simulink model "Senior_Design_G4"  (R2017b)
settings: Solver=ode3  StartTime=0.0  StopTime=inf  FixedStep=0.001  RelTol=1e-3  EnableMultiTasking=on
libraries: xpcquanserlib x5, slrtlib x2
settings Model: SimulationMode=external  Creator=Ninad  LastModifiedBy=basil
settings DataIOCC: LimitDataPoints=on  SaveFormat=Array
settings OptimizationCC: BlockReduction=off  OptimizeBlockIOStorage=off  BufferReuse=off  GlobalBufferReuse=off  ExpressionFolding=off  ExpressionDepthLimit=2147483647  LocalBlockOutputs=off  LifeSpan=inf
settings DebuggingCC: UnderspecifiedInitializationDetection=Classic  MergeDetectMultiDrivingBlocksExec=none  SolverPrmCheckMsg=warning  FcnCallInpInsideContextMsg=warning  StateNameClashWarn=warning  StrictBusMsg=Warning  SFUnexpectedBacktrackingDiag=warning  SFNoUnconditionalDefaultTransitionDiag=warning  SFExecutionAtInitializationDiag=none
settings HardwareCC: ProdBitPerPointer=32  ProdBitPerSizeT=32  ProdBitPerPtrDiffT=32  ProdLargestAtomicFloat=None  ProdWordSize=32  ProdLongLongMode=on  ProdHWDeviceType=Generic->32-bit x86 compatible
settings ModelReferenceCC: PropagateSignalLabelsOutOfModel=off
settings RTWCC: SystemTargetFile=slrt.tlc  TemplateMakefile=slrt_default_tmf  Description=Simulink Real-Time  CodeExecutionProfiling=on  RTWCompilerOptimization=on
settings CodeAppCC: StateflowObjectComments=on
settings SimulinkRealTimeCC: GeneratePreprocessorConditionals=Disable all
settings ConfigComp: CovMetricSettings=dw  CovHtmlReporting=on  CovSaveCumulativeToWorkspaceVar=on  CovSaveSingleToWorkspaceVar=on  CovExternalEMLEnable=off  CovSFcnEnable=off

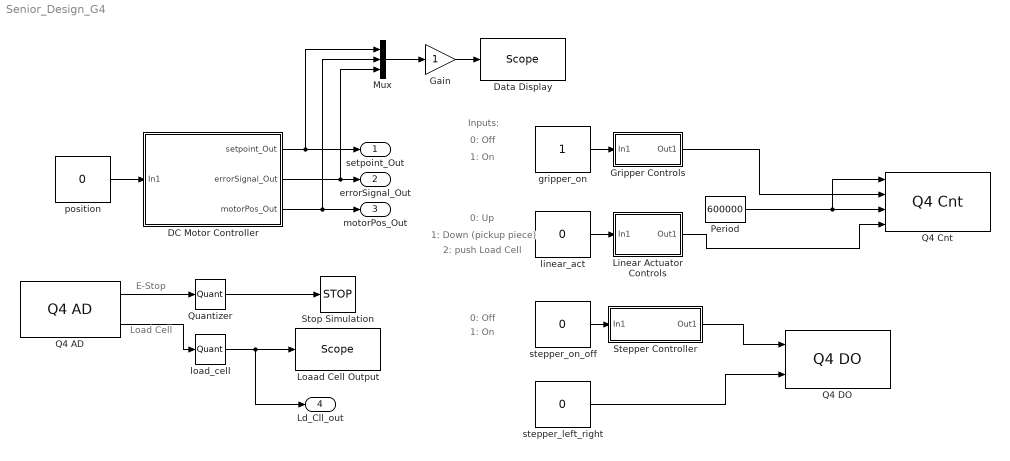
== system Senior_Design_G4 ==
  note: 1: On
  note: 0: Off
  note: 2: push Load Cell
  note: 1: Down (pickup piece)
  note: 0: Up
  note: 1: On
  note: 0: Off
  note: Inputs:
  note: Load Cell
  note: E-Stop
  DC Motor Controller : Subsystem
  Data Display : slrtlib/Displays and Logging/Scope   scopeno=1  scopetype=Target  autostart=on  viewmode=Numerical  formatstr="'Setpoint        %3.2f,Motor Position  %3.2f,Error Signal    %3.2f'"  grid=on  ylimits=[0,170]  nosamples=200  noprepostsamples=0  interleave=10  triggermode=FreeRun  triggersignal=1  trigsignalfromport=off  triggerlevel=0.0  triggerslope=Either  triggerscope=1  triggersample=0  filename=data.dat  mode=Lazy  writesize=512  autorestart=off  dynamicfilemode=off  maxwritefilesize=512*1024^2
  Gain : Gain
  Gripper Controls : Subsystem
  Linear Actuator Controls : Subsystem
  "Loaad Cell Output " : slrtlib/Displays and Logging/Scope   scopeno=4  scopetype=Target  autostart=on  viewmode=Graphical rolling  formatstr='%15.6f'  grid=on  ylimits=[-1,6]  nosamples=500  noprepostsamples=0  interleave=1  triggermode=FreeRun  triggersignal=1  trigsignalfromport=off  triggerlevel=0.0  triggerslope=Either  triggerscope=1  triggersample=0  filename=data.dat  mode=Lazy  writesize=512  autorestart=off  dynamicfilemode=off  maxwritefilesize=512*1024^2
  Mux : Mux  Inputs=3
  Period : Constant  Value=600000
  Q4 AD : xpcquanserlib/A//D/Q4 AD  channel=[1:2]  sampleTime=0.001  slot=-1
      settings: SourceProductName=Simulink Real-Time  SourceProductBaseCode=XP
  "Q4 Cnt " : xpcquanserlib/Counter/Q4 Cnt   channel=[1:2]  mode=[1]  showArm=[0]  reset=[1]  initLoCount=[0]  initHiCount=[0]  sampleTime=.001  slot=-1
      settings: SourceProductName=Simulink Real-Time  SourceProductBaseCode=XP
  "Q4 DO " : xpcquanserlib/Digital Output/Q4 DO   channel=[1:2]  reset=[1]  initValue=[0]  sampleTime=.001  slot=-1
      settings: SourceProductName=Simulink Real-Time  SourceProductBaseCode=XP
  Quantizer : Quantizer  QuantizationInterval=1
  Stepper Controller : Subsystem
  Stop Simulation : Stop
  gripper_on : Constant
  linear_act : Constant  Value=0
  load_cell : Quantizer  QuantizationInterval=5
  position : Constant  Value=0
  stepper_left_right : Constant  Value=0
  stepper_on_off : Constant  Value=0
  setpoint_Out : Outport
  errorSignal_Out : Outport  Port=2
  motorPos_Out : Outport  Port=3
  Ld_Cll_out : Outport  Port=4
  wires:
  Quantizer/1 -> Stop Simulation/1
  Q4 AD/1 -> Quantizer/1
  Q4 AD/2 -> load_cell/1
  load_cell/1 -> Ld_Cll_out/1, "Loaad Cell Output "/1
  Period/1 -> "Q4 Cnt "/1, "Q4 Cnt "/3
  stepper_left_right/1 -> "Q4 DO "/2
  DC Motor Controller/3(motorPos_Out) -> Mux/2, motorPos_Out/1
  position/1 -> DC Motor Controller/1(In1)
  gripper_on/1 -> Gripper Controls/1(In1)
  Gripper Controls/1(Out1) -> "Q4 Cnt "/2
  linear_act/1 -> Linear Actuator Controls/1(In1)
  Linear Actuator Controls/1(Out1) -> "Q4 Cnt "/4
  stepper_on_off/1 -> Stepper Controller/1(In1)
  Stepper Controller/1(Out1) -> "Q4 DO "/1
  Gain/1 -> Data Display/1
  DC Motor Controller/1(setpoint_Out) -> Mux/1, setpoint_Out/1
  DC Motor Controller/2(errorSignal_Out) -> Mux/3, errorSignal_Out/1
  Mux/1 -> Gain/1

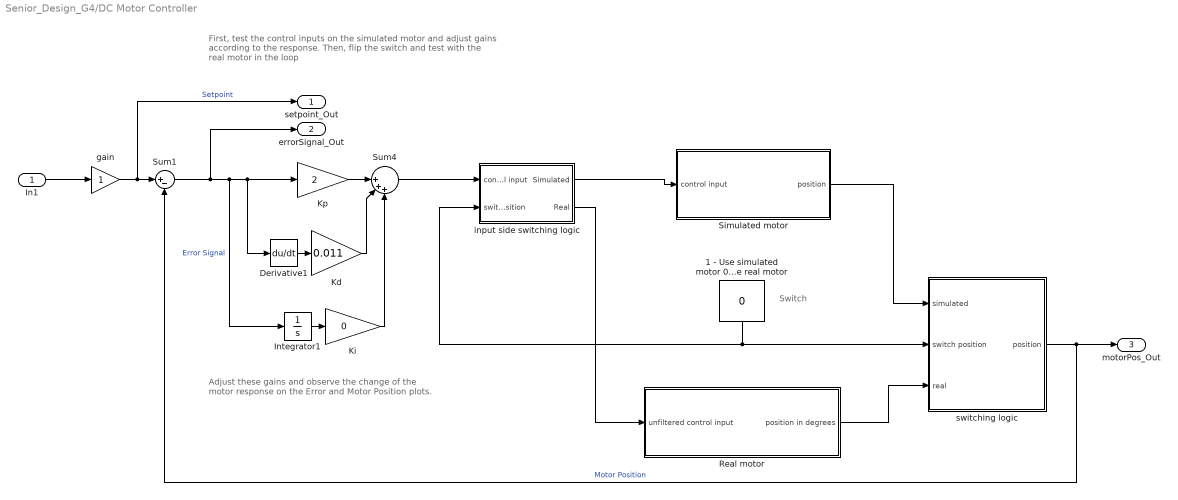
== system Senior_Design_G4/DC Motor Controller ==
  note: Adjust these gains and observe the change of the
      | motor response on the Error and Motor Position
      | plots.
  note: First, test the control inputs on the simulated motor and
      | adjust gains according to the response. Then, flip the switch and
      | test with the real motor in the loop
  note: Switch
  In1 : Inport
  1 - Use simulated motor 0 - Use real motor : Constant  Value=0
  Derivative1 : Derivative
  Integrator1 : Integrator
  Kd : Gain  Gain=0.011
  Ki : Gain  Gain=0
  Kp : Gain  Gain=2
  Real motor : Subsystem
  Simulated motor : Subsystem
  Sum1 : Sum  Inputs=|+-
  Sum4 : Sum  Inputs=||+++
  gain : Gain
  input side switching logic : Subsystem
  switching logic : Subsystem
  setpoint_Out : Outport
  errorSignal_Out : Outport  Port=2
  motorPos_Out : Outport  Port=3
  wires:
  Kp/1 -> Sum4/1
  Kd/1 -> Sum4/2
  Derivative1/1 -> Kd/1
  Ki/1 -> Sum4/3
  Integrator1/1 -> Ki/1
  Sum1/1 -> Kp/1, Derivative1/1, Integrator1/1, errorSignal_Out/1  "Error Signal"
  Simulated motor/1(position) -> switching logic/1(simulated)
  Real motor/1(position in degrees) -> switching logic/3(real)
  switching logic/1(position) -> motorPos_Out/1, Sum1/2  "Motor Position"
  Sum4/1 -> input side switching logic/1(control input)
  input side switching logic/1(Simulated) -> Simulated motor/1(control input)
  input side switching logic/2(Real) -> Real motor/1(unfiltered control input)
  1 - Use simulated motor 0 - Use real motor/1 -> switching logic/2(switch position), input side switching logic/2(switch position)
  In1/1 -> gain/1
  gain/1 -> Sum1/1, setpoint_Out/1  "Setpoint"

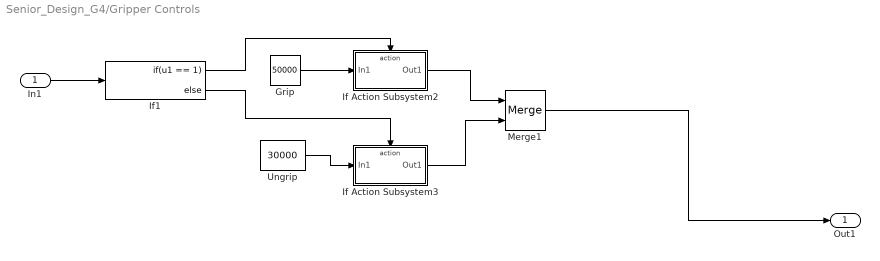
== system Senior_Design_G4/Gripper Controls ==
  In1 : Inport
  Grip : Constant  Value=50000
  If Action Subsystem2 : Subsystem  TreatAsAtomicUnit=on
  If Action Subsystem3 : Subsystem  TreatAsAtomicUnit=on
  If1 : If  IfExpression=u1 == 1
  Merge1 : Merge
  Ungrip : Constant  Value=30000
  Out1 : Outport
  wires:
  If Action Subsystem3/1(Out1) -> Merge1/2
  If Action Subsystem2/1(Out1) -> Merge1/1
  If1/2 -> If Action Subsystem3/Action
  Merge1/1 -> Out1/1
  If1/1 -> If Action Subsystem2/Action
  Grip/1 -> If Action Subsystem2/1(In1)
  In1/1 -> If1/1
  Ungrip/1 -> If Action Subsystem3/1(In1)

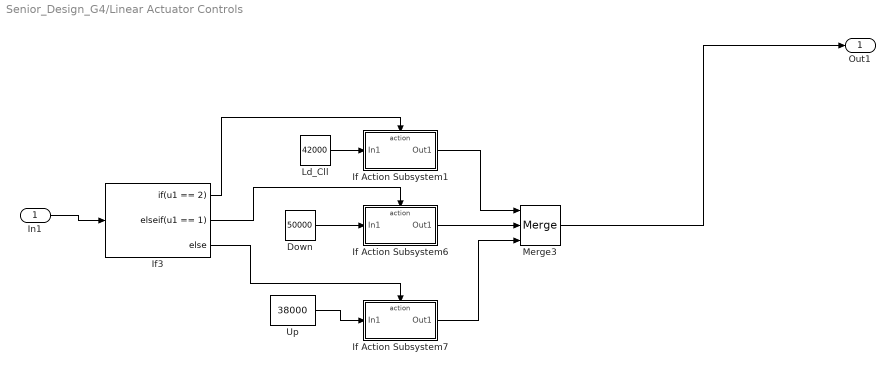
== system Senior_Design_G4/Linear Actuator Controls ==
  In1 : Inport
  Down : Constant  Value=50000
  If Action Subsystem1 : Subsystem  TreatAsAtomicUnit=on
  If Action Subsystem6 : Subsystem  TreatAsAtomicUnit=on
  If Action Subsystem7 : Subsystem  TreatAsAtomicUnit=on
  If3 : If  IfExpression=u1 == 2  ElseIfExpressions=u1 == 1
  Ld_Cll : Constant  Value=42000
  Merge3 : Merge  Inputs=3
  "Up " : Constant  Value=38000
  Out1 : Outport
  wires:
  If Action Subsystem7/1(Out1) -> Merge3/3
  Ld_Cll/1 -> If Action Subsystem1/1(In1)
  "Up "/1 -> If Action Subsystem7/1(In1)
  If3/1 -> If Action Subsystem1/Action
  If3/2 -> If Action Subsystem6/Action
  If3/3 -> If Action Subsystem7/Action
  Down/1 -> If Action Subsystem6/1(In1)
  If Action Subsystem1/1(Out1) -> Merge3/1
  In1/1 -> If3/1
  Merge3/1 -> Out1/1
  If Action Subsystem6/1(Out1) -> Merge3/2

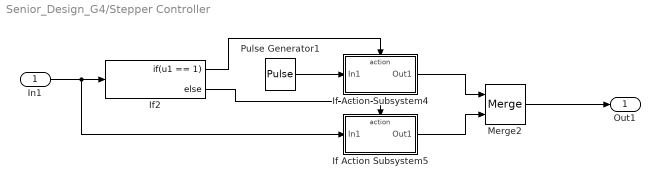
== system Senior_Design_G4/Stepper Controller ==
  In1 : Inport
  If Action Subsystem4 : Subsystem  TreatAsAtomicUnit=on
  If Action Subsystem5 : Subsystem  TreatAsAtomicUnit=on
  If2 : If  IfExpression=u1 == 1
  Merge2 : Merge
  Pulse Generator1 : DiscretePulseGenerator  PulseType=Time based  Amplitude=5  Period=0.01  PulseWidth=50
  Out1 : Outport
  wires:
  In1/1 -> If Action Subsystem5/1(In1), If2/1
  If2/1 -> If Action Subsystem4/Action
  If Action Subsystem4/1(Out1) -> Merge2/1
  If Action Subsystem5/1(Out1) -> Merge2/2
  Merge2/1 -> Out1/1
  Pulse Generator1/1 -> If Action Subsystem4/1(In1)
  If2/2 -> If Action Subsystem5/Action

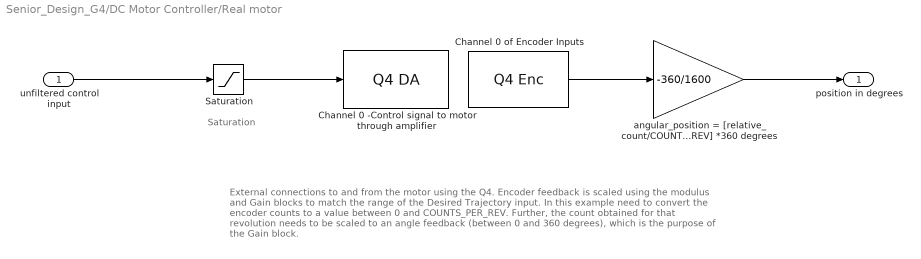
== system Senior_Design_G4/DC Motor Controller/Real motor ==
  note: Saturation
  note: External connections to and from the motor using the Q4.
      |
      | Encoder feedback is scaled using the modulus and Gain blocks to
      | match the range of the Desired Trajectory input.
      |
      | In this example need to convert the encoder counts to a value between 0 and COUNTS_PER_REV.
      | Further, the count obtained for that revolution needs to be scaled to an angle feedback (between
      | 0 and 360 degrees), which is the purpose of the Gain block.
  unfiltered control input : Inport
  "Channel 0 -Control signal to motor through amplifier " : xpcquanserlib/D//A/Q4 DA   channel=[1]  range=[-10]  simul=off  reset=[1]  initValue=[0]  sampleTime=.001  slot=-1
      settings: SourceProductName=Simulink Real-Time  SourceProductBaseCode=XP
  "Channel 0 of Encoder Inputs " : xpcquanserlib/Incremental Encoder/Q4 Enc   channel=[1]  initialCount=[0]  prescale=[1]  quadrature=[4]  mode=[0]  synchronousIndex=[0]  indexPolarity=[0]  preserveCounts=[0]  sampleTime=.001  slot=-1
      settings: SourceProductName=Simulink Real-Time  SourceProductBaseCode=XP
  Saturation : Saturate  UpperLimit=4  LowerLimit=-4
  angular_position = [relative_count/COUNTS_PER_REV] *360 degrees : Gain  Gain=-360/1600
  position in degrees : Outport
  wires:
  Saturation/1 -> "Channel 0 -Control signal to motor through amplifier "/1
  angular_position = [relative_count/COUNTS_PER_REV] *360 degrees/1 -> position in degrees/1
  "Channel 0 of Encoder Inputs "/1 -> angular_position = [relative_count/COUNTS_PER_REV] *360 degrees/1
  unfiltered control input/1 -> Saturation/1

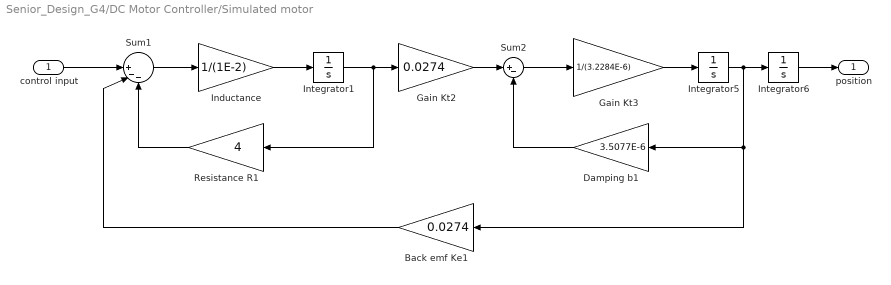
== system Senior_Design_G4/DC Motor Controller/Simulated motor ==
  control input : Inport
  Back emf Ke1 : Gain  Gain=0.0274
  Damping b1 : Gain  Gain=3.5077E-6
  Gain Kt2 : Gain  Gain=0.0274
  Gain Kt3 : Gain  Gain=1/(3.2284E-6)
  Inductance : Gain  Gain=1/(1E-2)
  Integrator1 : Integrator
  Integrator5 : Integrator
  Integrator6 : Integrator
  Resistance R1 : Gain  Gain=4
  Sum1 : Sum  Inputs=||+--
  Sum2 : Sum  Inputs=|+-
  position : Outport
  wires:
  Sum1/1 -> Inductance/1
  Inductance/1 -> Integrator1/1
  Integrator1/1 -> Gain Kt2/1, Resistance R1/1
  Gain Kt2/1 -> Sum2/1
  Sum2/1 -> Gain Kt3/1
  Gain Kt3/1 -> Integrator5/1
  Integrator5/1 -> Integrator6/1, Back emf Ke1/1, Damping b1/1
  Back emf Ke1/1 -> Sum1/2
  Damping b1/1 -> Sum2/2
  Resistance R1/1 -> Sum1/3
  Integrator6/1 -> position/1
  control input/1 -> Sum1/1

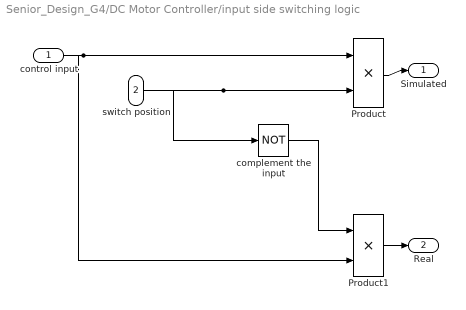
== system Senior_Design_G4/DC Motor Controller/input side switching logic ==
  control input : Inport
  switch position : Inport  Port=2
  Product : Product  RndMeth=Zero
  Product1 : Product  RndMeth=Zero
  complement the input : Logic  Operator=NOT  AllPortsSameDT=off  OutDataTypeStr=boolean
  Simulated : Outport
  Real : Outport  Port=2
  wires:
  control input/1 -> Product1/2, Product/1
  complement the input/1 -> Product1/1
  switch position/1 -> complement the input/1, Product/2
  Product/1 -> Simulated/1
  Product1/1 -> Real/1

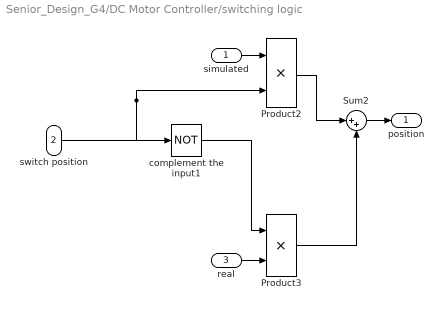
== system Senior_Design_G4/DC Motor Controller/switching logic ==
  simulated : Inport
  switch position : Inport  Port=2
  real : Inport  Port=3
  Product2 : Product  RndMeth=Zero
  Product3 : Product  RndMeth=Zero
  Sum2 : Sum  Inputs=|++
  complement the input1 : Logic  Operator=NOT  AllPortsSameDT=off  OutDataTypeStr=boolean
  position : Outport
  wires:
  complement the input1/1 -> Product3/1
  Product2/1 -> Sum2/1
  Product3/1 -> Sum2/2
  switch position/1 -> complement the input1/1, Product2/2
  simulated/1 -> Product2/1
  Sum2/1 -> position/1
  real/1 -> Product3/2

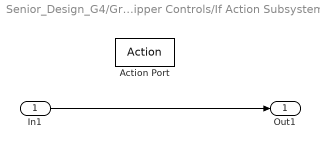
== system Senior_Design_G4/Gripper Controls/If Action Subsystem2 ==
  In1 : Inport
  Action Port : ActionPort  ActionType=then
  Out1 : Outport
  wires:
  In1/1 -> Out1/1

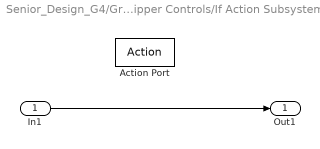
== system Senior_Design_G4/Gripper Controls/If Action Subsystem3 ==
  In1 : Inport
  Action Port : ActionPort  ActionType=else
  Out1 : Outport
  wires:
  In1/1 -> Out1/1

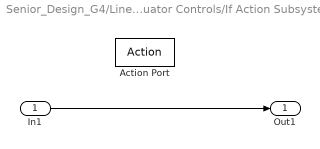
== system Senior_Design_G4/Linear Actuator Controls/If Action Subsystem1 ==
  In1 : Inport
  Action Port : ActionPort  ActionType=then
  Out1 : Outport
  wires:
  In1/1 -> Out1/1

== system Senior_Design_G4/Linear Actuator Controls/If Action Subsystem6 ==
  In1 : Inport
  Action Port : ActionPort  ActionType=elseif
  Out1 : Outport
  wires:
  In1/1 -> Out1/1

== system Senior_Design_G4/Linear Actuator Controls/If Action Subsystem7 ==
  In1 : Inport
  Action Port : ActionPort  ActionType=else
  Out1 : Outport
  wires:
  In1/1 -> Out1/1

== system Senior_Design_G4/Stepper Controller/If Action Subsystem4 ==
  In1 : Inport
  Action Port : ActionPort  ActionType=then
  Out1 : Outport
  wires:
  In1/1 -> Out1/1

== system Senior_Design_G4/Stepper Controller/If Action Subsystem5 ==
  In1 : Inport
  Action Port : ActionPort  ActionType=else
  Out1 : Outport
  wires:
  In1/1 -> Out1/1
